simulink model "Proj4_simulink"  (R2023b)
settings: Solver=FixedStepAuto  StartTime=0.0  StopTime=10  FixedStep=0.01  RelTol=1e-3
values from neighbouring files (symbols this model uses):
  test_position = [test_position, x]    [Proj4_MainScript.m]
  test_speed = [test_speed,20]    [Proj4_MainScript.m]
  x_track = [x_straight1, x_curve1, x_straight2, x_curve2]    [Proj4_MainScript.m]
  y_track = [y_straight1, y_curve1, y_straight2, y_curve2]    [Proj4_MainScript.m]
undefined symbols (not defined in the file or in its folder): batData, carData, motorData, mph2mps
libraries: slpidlib x2
settings Model: Creator=nakro  LastModifiedBy=nakro

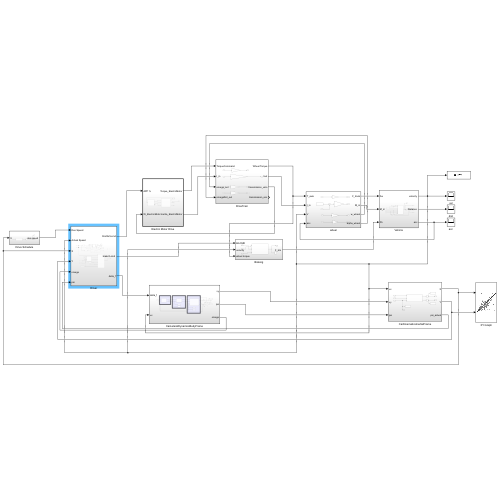
[thumbnail: Simulink's stored preview of the top-level diagram]
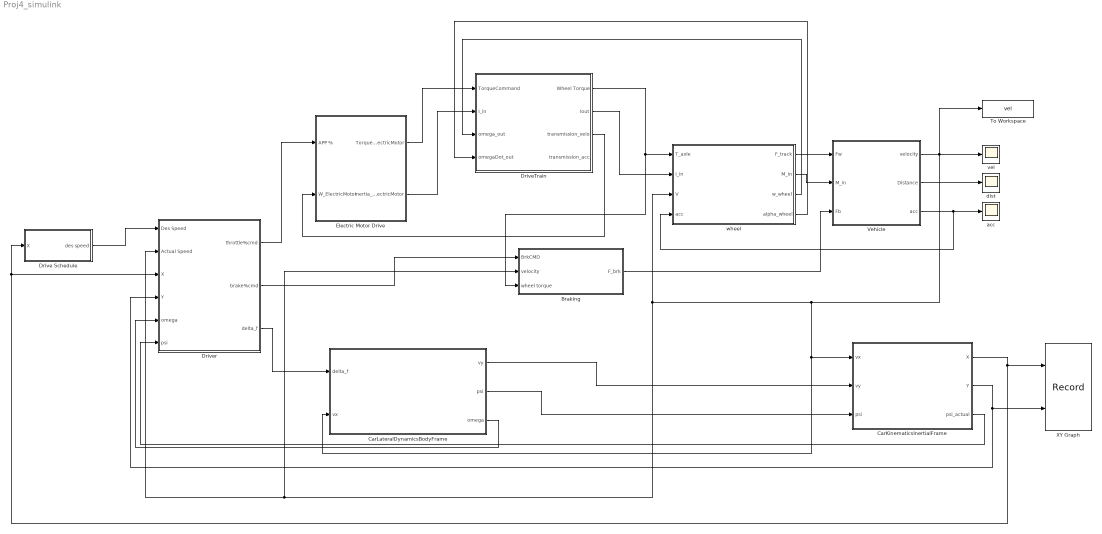
== system Proj4_simulink ==
  Braking : Subsystem
  CarKinematicsInertialFrame : Subsystem
  CarLateralDynamicsBodyFrame : Subsystem
  Drive Schedule : Subsystem
  DriveTrain : Subsystem
  "Driver " : Subsystem
  Electric Motor Drive : Subsystem  TreatAsAtomicUnit=on
  To Workspace : ToWorkspace  VariableName=vel  SaveFormat=Timeseries  SampleTime=0.01
  Vehicle : Subsystem
  XY Graph : Record  FileSettingsInternal="{\"entries\":[{\"content\":{\"excelSettings\":{\"content\":{},\"type\":\"Streamout.ExcelSettings\"}},\"type\":\"Streamout.FileSettingStorage\",\"uuid\":\"\"}],\"packageUris\":[\"http:\\/\\/schema.mathworks.com\\/mf0\\/streamout_blocks\\/R2020a\"],\"version\":\"1.0\"}"  Layout=[1 1]  SignalsInternal="{\"entries\":[{\"content\":{\"signals\":[{\"content\":{\"blockPath\":[],\"dimensions\":[1],\"domain\":\"\",\"lineColor\":\"#a2142f\",\"plots\":[1],\"port\":1,\"sid\":[\"\"],\"signalID\":43985,\"signalName\":\"CarKinematicsInertialFrame:1\"},\"type\":\"RecordBlkView.Signal\",\"uuid\":\"\"},{\"content\":{\"blockPath\":[],\"dimensions\":[1],\"domain\":\"\",\"lineColor\":\"#139fff\",\"plots\":[1],\"port\":2,\"sid\":[\"\"],\"signalID\":43989,\"signalName\":\"CarKinematicsInertialFrame:2\"},\"type\":\"RecordBlkView.Signal\",\"uuid\":\"\"}]},\"type\":\"RecordBlkView.InputSignals\",\"uuid\":\"\"}],\"packageUris\":[\"http:\\/\\/schema.mathworks.com\\/mf0\\/streamout_blocks\\/R2020a\"],\"version\":\"1.0\"}"  VisualizationBindings="{\"xyplotplugin\":{\"info\":[{\"series\":[{\"bindingParametersList\":[{\"parameter\":\"X-Axis\",\"signalID\":43985,\"signalName\":\"CarKinematicsInertialFrame:1\"},{\"parameter\":\"Y-Axis\",\"signalID\":43989,\"signalName\":\"CarKinematicsInertialFrame:2\"}],\"seriesID\":61081}],\"subplotID\":1}]}}"  CompatibilityTag=XY  st=-1
  acc : Scope
  dist : Scope
  vel : Scope
  "wheel " : Subsystem
  wires:
  CarLateralDynamicsBodyFrame/2(psi) -> CarKinematicsInertialFrame/3(psi)
  CarKinematicsInertialFrame/1(X) -> "Driver "/3(X), Drive Schedule/1(X), XY Graph/1
  CarLateralDynamicsBodyFrame/1(vy) -> CarKinematicsInertialFrame/2(vy)
  CarKinematicsInertialFrame/2(Y) -> XY Graph/2, "Driver "/4(Y)
  Electric Motor Drive/1(Torque_ElectricMotor) -> DriveTrain/1(TorqueCommand)
  Vehicle/1("velocity ") -> Braking/2("velocity "), "Driver "/2(Actual Speed), "wheel "/3(V), CarKinematicsInertialFrame/1(vx), CarLateralDynamicsBodyFrame/2(vx), To Workspace/1, vel/1
  Electric Motor Drive/2(Inertia_ElectricMotor) -> DriveTrain/2(I_in)
  "wheel "/3(w_wheel) -> DriveTrain/3(omega_out)
  "Driver "/1(throttle%cmd) -> Electric Motor Drive/1(APP %)
  "wheel "/4(alpha_wheel) -> DriveTrain/4(omegaDot_out)
  "wheel "/1(F_track) -> Vehicle/1("Fw ")
  Vehicle/2("Distance ") -> dist/1
  DriveTrain/1(Wheel Torque) -> Braking/3(wheel torque), "wheel "/1(T_axle)
  Vehicle/3(acc) -> acc/1, "wheel "/4(acc)
  DriveTrain/3(transmission_velo) -> Electric Motor Drive/2(W_ElectricMotor)
  "wheel "/2(M_in) -> Vehicle/2("M_in ")
  Braking/1("F_brk ") -> Vehicle/3("Fb ")
  Drive Schedule/1("des speed ") -> "Driver "/1("Des Speed ")
  DriveTrain/2(Iout) -> "wheel "/2(I_in)
  "Driver "/2("brake%cmd ") -> Braking/1("BrkCMD ")
  "Driver "/3(delta_f) -> CarLateralDynamicsBodyFrame/1(delta_f)
  CarKinematicsInertialFrame/3(psi_actual) -> "Driver "/6(psi)
  CarLateralDynamicsBodyFrame/3(omega) -> "Driver "/5(omega)

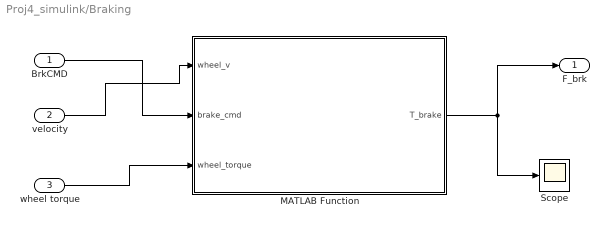
== system Proj4_simulink/Braking ==
  "BrkCMD " : Inport
  "velocity " : Inport  Port=2
  wheel torque : Inport  Port=3
  MATLAB Function : MATLAB Function  TreatAsAtomicUnit=on
  Scope : Scope
  "F_brk " : Outport  VectorParamsAs1DForOutWhenUnconnected=off
  wires:
  "BrkCMD "/1 -> MATLAB Function/2(brake_cmd)
  "velocity "/1 -> MATLAB Function/1(wheel_v)
  wheel torque/1 -> MATLAB Function/3(wheel_torque)
  MATLAB Function/1(T_brake) -> Scope/1, "F_brk "/1

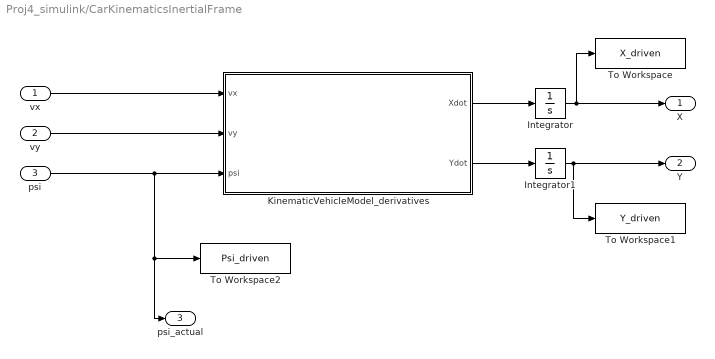
== system Proj4_simulink/CarKinematicsInertialFrame ==
  vx : Inport
  vy : Inport  Port=2
  psi : Inport  Port=3
  Integrator : Integrator  InitialCondition=carData.init.X0
  Integrator1 : Integrator  InitialCondition=carData.init.Y0
  KinematicVehicleModel_derivatives : MATLAB Function  TreatAsAtomicUnit=on  mask{obj=carData}
      mask prompts: obj "obj structure"
  To Workspace : ToWorkspace  VariableName=X_driven  SaveFormat=Timeseries  SampleTime=0.1
  To Workspace1 : ToWorkspace  VariableName=Y_driven  SaveFormat=Timeseries  SampleTime=0.1
  To Workspace2 : ToWorkspace  VariableName=Psi_driven  SaveFormat=Timeseries  SampleTime=0.1
  X : Outport
  Y : Outport  Port=2
  psi_actual : Outport  Port=3
  wires:
  KinematicVehicleModel_derivatives/1(Xdot) -> Integrator/1
  KinematicVehicleModel_derivatives/2(Ydot) -> Integrator1/1
  Integrator/1 -> To Workspace/1, X/1
  Integrator1/1 -> To Workspace1/1, Y/1
  vx/1 -> KinematicVehicleModel_derivatives/1(vx)
  vy/1 -> KinematicVehicleModel_derivatives/2(vy)
  psi/1 -> psi_actual/1, To Workspace2/1, KinematicVehicleModel_derivatives/3(psi)

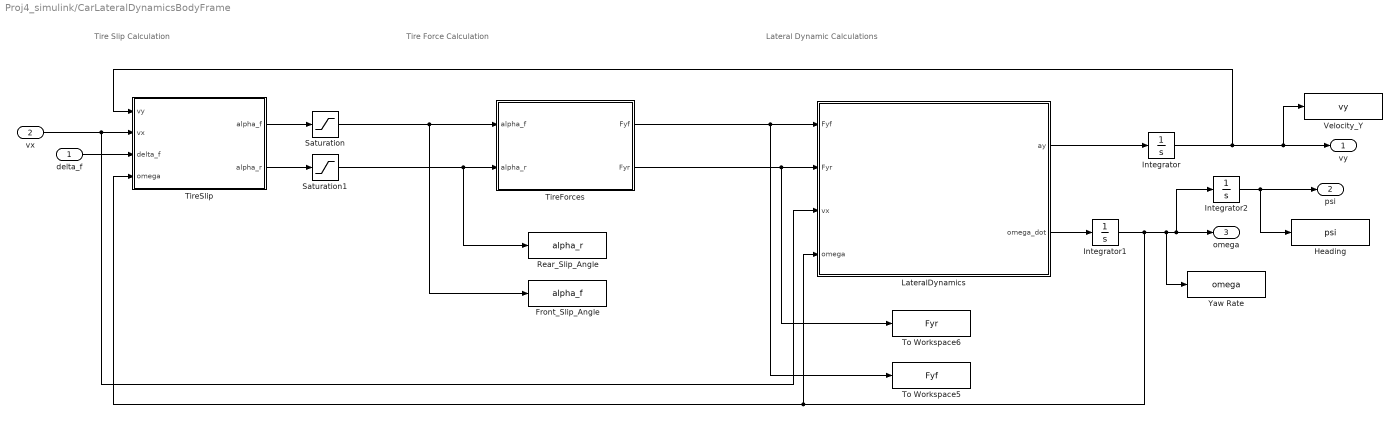
== system Proj4_simulink/CarLateralDynamicsBodyFrame ==
  note: Tire Slip Calculation
  note: Tire Force Calculation
  note: Lateral Dynamic Calculations
  delta_f : Inport
  vx : Inport  Port=2
  Front_Slip_Angle : ToWorkspace  VariableName=alpha_f  SaveFormat=Timeseries  SampleTime=0.01
  Heading : ToWorkspace  VariableName=psi  SaveFormat=Timeseries  SampleTime=0.01
  Integrator : Integrator  InitialCondition=carData.init.vy0
  Integrator1 : Integrator  InitialCondition=carData.init.omega0
  Integrator2 : Integrator  InitialCondition=carData.init.psi0
  LateralDynamics : MATLAB Function  TreatAsAtomicUnit=on  mask{obj=carData}
      mask prompts: obj "obj structure"
  Rear_Slip_Angle : ToWorkspace  VariableName=alpha_r  SaveFormat=Timeseries  SampleTime=0.01
  Saturation : Saturate  UpperLimit=carData.maxAlpha  LowerLimit=-carData.maxAlpha
  Saturation1 : Saturate  UpperLimit=carData.maxAlpha  LowerLimit=-carData.maxAlpha
  TireForces : MATLAB Function  TreatAsAtomicUnit=on  mask{obj=carData}
      mask prompts: obj "obj structure"
  TireSlip : MATLAB Function  TreatAsAtomicUnit=on  mask{obj=carData}
      mask prompts: obj "obj structure"
  To Workspace5 : ToWorkspace  VariableName=Fyf  SaveFormat=Timeseries  SampleTime=0.01
  To Workspace6 : ToWorkspace  VariableName=Fyr  SaveFormat=Timeseries  SampleTime=0.01
  Velocity_Y : ToWorkspace  VariableName=vy  SaveFormat=Timeseries  SampleTime=0.01
  Yaw Rate : ToWorkspace  VariableName=omega  SaveFormat=Timeseries  SampleTime=0.01
  vy : Outport
  psi : Outport  Port=2
  omega : Outport  Port=3
  wires:
  LateralDynamics/1(ay) -> Integrator/1
  Integrator/1 -> vy/1, Velocity_Y/1, TireSlip/1(vy)
  LateralDynamics/2(omega_dot) -> Integrator1/1
  Integrator1/1 -> Integrator2/1, omega/1, Yaw Rate/1, LateralDynamics/4(omega), TireSlip/4(omega)
  TireSlip/1(alpha_f) -> Saturation/1
  TireSlip/2(alpha_r) -> Saturation1/1
  TireForces/1(Fyf) -> LateralDynamics/1(Fyf), To Workspace5/1
  TireForces/2(Fyr) -> LateralDynamics/2(Fyr), To Workspace6/1
  Saturation/1 -> TireForces/1(alpha_f), Front_Slip_Angle/1
  Saturation1/1 -> TireForces/2(alpha_r), Rear_Slip_Angle/1
  vx/1 -> TireSlip/2(vx), LateralDynamics/3(vx)
  delta_f/1 -> TireSlip/3(delta_f)
  Integrator2/1 -> Heading/1, psi/1

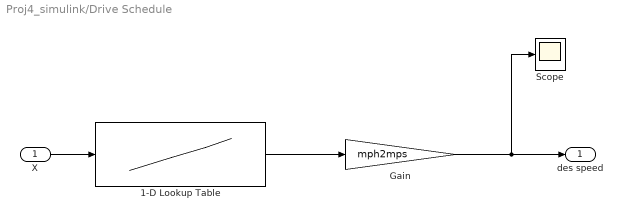
== system Proj4_simulink/Drive Schedule ==
  X : Inport
  1-D Lookup Table : Lookup_n-D  NumberOfTableDimensions=1  BreakpointsForDimension1=test_position  Table=test_speed  InternalRulePriority=Speed  RndMeth=Simplest
  Gain : Gain  Gain=mph2mps
  Scope : Scope
  "des speed " : Outport  VectorParamsAs1DForOutWhenUnconnected=off
  wires:
  1-D Lookup Table/1 -> Gain/1
  Gain/1 -> "des speed "/1, Scope/1
  X/1 -> 1-D Lookup Table/1

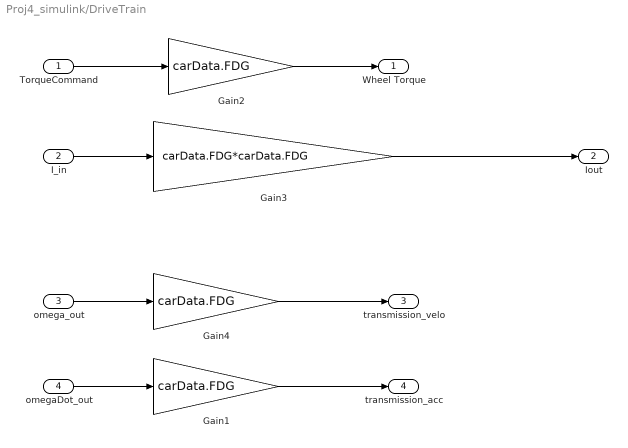
== system Proj4_simulink/DriveTrain ==
  TorqueCommand : Inport
  I_in : Inport  Port=2
  omega_out : Inport  Port=3
  omegaDot_out : Inport  Port=4
  Gain1 : Gain  Gain=carData.FDG
  Gain2 : Gain  Gain=carData.FDG
  Gain3 : Gain  Gain=carData.FDG*carData.FDG
  Gain4 : Gain  Gain=carData.FDG
  Wheel Torque : Outport
  Iout : Outport  Port=2
  transmission_velo : Outport  Port=3
  transmission_acc : Outport  Port=4
  wires:
  Gain4/1 -> transmission_velo/1
  Gain3/1 -> Iout/1
  Gain1/1 -> transmission_acc/1
  Gain2/1 -> Wheel Torque/1
  TorqueCommand/1 -> Gain2/1
  omega_out/1 -> Gain4/1
  omegaDot_out/1 -> Gain1/1
  I_in/1 -> Gain3/1

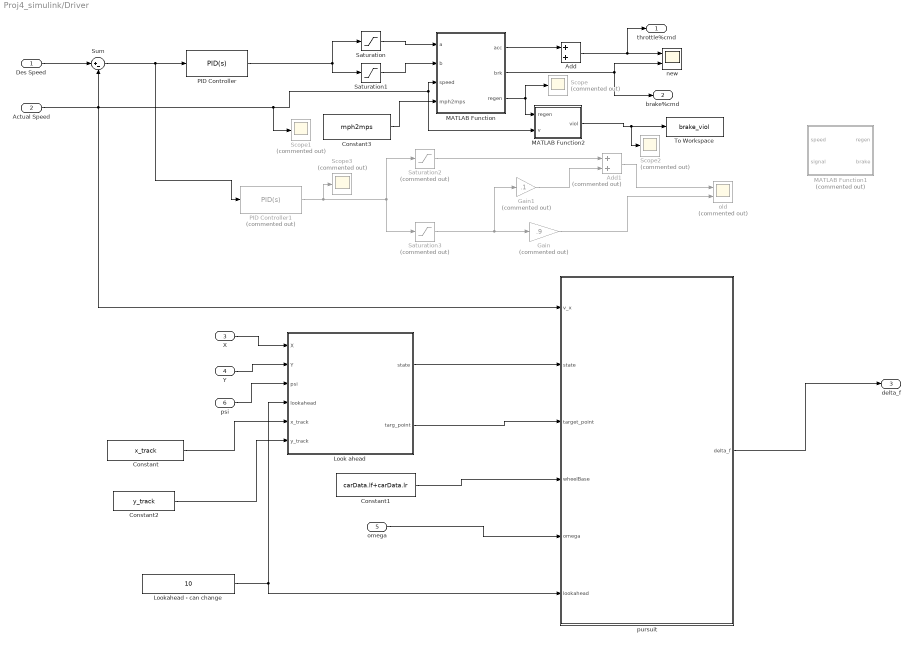
== system Proj4_simulink/Driver  ==
  "Des Speed " : Inport
  Actual Speed : Inport  Port=2
  X : Inport  Port=3
  Y : Inport  Port=4
  omega : Inport  Port=5
  psi : Inport  Port=6
  Add : Sum
  Add1 : Sum  Commented=on
  Constant : Constant  Value=x_track
  Constant1 : Constant  Value=carData.lf+carData.lr
  Constant2 : Constant  Value=y_track
  Constant3 : Constant  Value=mph2mps
  Gain : Gain  Commented=on  Gain=.9
  Gain1 : Gain  Commented=on  Gain=.1
  Look ahead : MATLAB Function  TreatAsAtomicUnit=on
  Lookahead - can change : Constant  Value=10
  MATLAB Function : MATLAB Function  TreatAsAtomicUnit=on
  MATLAB Function1 : MATLAB Function  Commented=on  TreatAsAtomicUnit=on
  MATLAB Function2 : MATLAB Function  TreatAsAtomicUnit=on
  PID Controller : slpidlib/PID Controller  Controller=PID  Form=Parallel  TimeDomain=Continuous-time  UseExternalTs=on  SampleTime=0.01  IntegratorMethod=Forward Euler  FilterMethod=Forward Euler  ControllerParametersSource=internal  P=.1  I=0  UseKiTs=off  D=0  N=100  UseFilter=on  TunerSelectOption=Transfer Function Based (PID Tuner App)  InitialConditionSource=internal  InitialConditionForIntegrator=0  InitialConditionForFilter=0  DifferentiatorICPrevScaledInput=0  ExternalReset=none  TrackingMode=off  Kt=1  LimitOutput=on  SatLimitsSource=internal  UpperSaturationLimit=1  LowerSaturationLimit=-1  LinearizeAsGain=off  AntiWindupMode=none  Kb=1  LimitIntegrator=off  UpperIntegratorSaturationLimit=inf  LowerIntegratorSaturationLimit=-inf  POutMin=[]  POutMax=[]  IOutMin=[]  IOutMax=[]  DOutMin=[]  DOutMax=[]  NOutMin=[]  NOutMax=[]  SumOutMin=[]  SumOutMax=[]  SaturationOutMin=[]  SaturationOutMax=[]  PParamMin=[]  PParamMax=[]  IParamMin=[]  IParamMax=[]  DParamMin=[]  DParamMax=[]  NParamMin=[]  NParamMax=[]  KbParamMin=[]  KbParamMax=[]  KtParamMin=[]  KtParamMax=[]  KbOutMin=[]  KbOutMax=[]  KtOutMin=[]  KtOutMax=[]  IntegratorOutMin=[]  IntegratorOutMax=[]  FilterOutMin=[]  FilterOutMax=[]  SumI1OutMin=[]  SumI1OutMax=[]  SumI2OutMin=[]  SumI2OutMax=[]  SumI3OutMin=[]  SumI3OutMax=[]  SumI4OutMin=[]  SumI4OutMax=[]  SumDOutMin=[]  SumDOutMax=[]  DifferentiatorOutMin=[]  DifferentiatorOutMax=[]  FilterDiffOutCoefMin=[]  FilterDiffOutCoefMax=[]  ReciprocalOutMin=[]  ReciprocalOutMax=[]  SumDenOutMin=[]  SumDenOutMax=[]  SumNumOutMin=[]  SumNumOutMax=[]  DivideOutMin=[]  DivideOutMax=[]  UdiffTsProdOutMin=[]  UdiffTsProdOutMax=[]  NTsProdOutMin=[]  NTsProdOutMax=[]  UintegralTsProdOutMin=[]  UintegralTsProdOutMax=[]  UngainTsProdOutMin=[]  UngainTsProdOutMax=[]  ClampingZeroOutDataTypeStr=Inherit: Inherit via back propagation  ClampingZeroOutMin=[]  ClampingZeroOutMax=[]  FilterDenConstantOutDataTypeStr=Inherit: Inherit via back propagation  FilterDenConstantOutMin=[]  FilterDenConstantOutMax=[]  PCopyOutDataTypeStr=Inherit: Inherit via back propagation  PCopyOutMin=[]  PCopyOutMax=[]  NCopyOutDataTypeStr=Inherit: Inherit via back propagation  NCopyOutMin=[]  NCopyOutMax=[]  IntegratorContinuousStateAttributes=''  IntegratorStateMustResolveToSignalObject=off  IntegratorRTWStateStorageClass=Auto  FilterContinuousStateAttributes=''  FilterStateMustResolveToSignalObject=off  FilterRTWStateStorageClass=Auto  ParallelPVariant=InternalParameters  IdealPVariant=Disabled  IVariant=InternalParameters  DVariant=InternalParameters  IntegratorVariant=Continuous  SatVariant=Enabled  AWVariant=Passthrough  PCopyVariant=Disabled  TRVariant=Disabled  FdbkBlocksVariant=Forward  IdealPFdbkVariant=Disabled  SatFdbkVariant=Disabled  DerivativeFilterVariant=ContFilter  NVariant=InternalParameters  NCopyVariant=Disabled  FilterICVariant=InternalICsFilter  IntegratorICVariant=InternalICs  ExternalResetVariant=Disabled  TRSumVariant=Passthrough  SumFdbkVariant=Disabled  SumVariant=Sum_PID  TsampFilterVariant=InternalTs  TsampNgainVariant=Passthrough  TsampIntegralVariant=Disabled_SignalSpec  ExternalSaturationOutDataTypeStr=Inherit: Same as second input
  PID Controller1 : slpidlib/PID Controller  Commented=on  Controller=PID  Form=Parallel  TimeDomain=Continuous-time  UseExternalTs=off  SampleTime=-1  IntegratorMethod=Forward Euler  FilterMethod=Forward Euler  ControllerParametersSource=internal  P=.1  I=0  UseKiTs=off  D=0  N=100  UseFilter=on  TunerSelectOption=Transfer Function Based (PID Tuner App)  InitialConditionSource=internal  InitialConditionForIntegrator=0  InitialConditionForFilter=0  DifferentiatorICPrevScaledInput=0  ExternalReset=none  TrackingMode=off  Kt=1  LimitOutput=on  SatLimitsSource=internal  UpperSaturationLimit=1  LowerSaturationLimit=-1  LinearizeAsGain=off  AntiWindupMode=none  Kb=1  LimitIntegrator=off  UpperIntegratorSaturationLimit=inf  LowerIntegratorSaturationLimit=-inf  POutMin=[]  POutMax=[]  IOutMin=[]  IOutMax=[]  DOutMin=[]  DOutMax=[]  NOutMin=[]  NOutMax=[]  SumOutMin=[]  SumOutMax=[]  SaturationOutMin=[]  SaturationOutMax=[]  PParamMin=[]  PParamMax=[]  IParamMin=[]  IParamMax=[]  DParamMin=[]  DParamMax=[]  NParamMin=[]  NParamMax=[]  KbParamMin=[]  KbParamMax=[]  KtParamMin=[]  KtParamMax=[]  KbOutMin=[]  KbOutMax=[]  KtOutMin=[]  KtOutMax=[]  IntegratorOutMin=[]  IntegratorOutMax=[]  FilterOutMin=[]  FilterOutMax=[]  SumI1OutMin=[]  SumI1OutMax=[]  SumI2OutMin=[]  SumI2OutMax=[]  SumI3OutMin=[]  SumI3OutMax=[]  SumI4OutMin=[]  SumI4OutMax=[]  SumDOutMin=[]  SumDOutMax=[]  DifferentiatorOutMin=[]  DifferentiatorOutMax=[]  FilterDiffOutCoefMin=[]  FilterDiffOutCoefMax=[]  ReciprocalOutMin=[]  ReciprocalOutMax=[]  SumDenOutMin=[]  SumDenOutMax=[]  SumNumOutMin=[]  SumNumOutMax=[]  DivideOutMin=[]  DivideOutMax=[]  UdiffTsProdOutMin=[]  UdiffTsProdOutMax=[]  NTsProdOutMin=[]  NTsProdOutMax=[]  UintegralTsProdOutMin=[]  UintegralTsProdOutMax=[]  UngainTsProdOutMin=[]  UngainTsProdOutMax=[]  ClampingZeroOutDataTypeStr=Inherit: Inherit via back propagation  ClampingZeroOutMin=[]  ClampingZeroOutMax=[]  FilterDenConstantOutDataTypeStr=Inherit: Inherit via back propagation  FilterDenConstantOutMin=[]  FilterDenConstantOutMax=[]  PCopyOutDataTypeStr=Inherit: Inherit via back propagation  PCopyOutMin=[]  PCopyOutMax=[]  NCopyOutDataTypeStr=Inherit: Inherit via back propagation  NCopyOutMin=[]  NCopyOutMax=[]  IntegratorContinuousStateAttributes=''  IntegratorStateMustResolveToSignalObject=off  IntegratorRTWStateStorageClass=Auto  FilterContinuousStateAttributes=''  FilterStateMustResolveToSignalObject=off  FilterRTWStateStorageClass=Auto  ParallelPVariant=InternalParameters  IdealPVariant=Disabled  IVariant=InternalParameters  DVariant=InternalParameters  IntegratorVariant=Continuous  SatVariant=Enabled  AWVariant=Passthrough  PCopyVariant=Disabled  TRVariant=Disabled  FdbkBlocksVariant=Forward  IdealPFdbkVariant=Disabled  SatFdbkVariant=Disabled  DerivativeFilterVariant=ContFilter  NVariant=InternalParameters  NCopyVariant=Disabled  FilterICVariant=InternalICsFilter  IntegratorICVariant=InternalICs  ExternalResetVariant=Disabled  TRSumVariant=Passthrough  SumFdbkVariant=Disabled  SumVariant=Sum_PID  TsampFilterVariant=InternalTs  TsampNgainVariant=Passthrough  TsampIntegralVariant=Disabled_SignalSpec  ExternalSaturationOutDataTypeStr=Inherit: Same as second input
  Saturation : Saturate  UpperLimit=1  LowerLimit=0
  Saturation1 : Saturate  UpperLimit=0  LowerLimit=-1
  Saturation2 : Saturate  Commented=on  UpperLimit=1  LowerLimit=0
  Saturation3 : Saturate  Commented=on  UpperLimit=0  LowerLimit=-1
  Scope{,1..3} (4 alike) : Scope  Commented=on
  Sum : Sum  Inputs=|+-
  To Workspace : ToWorkspace  VariableName=brake_viol  SaveFormat=Timeseries  SampleTime=0.01
  new : Scope  NumInputPorts=2
  old : Scope  Commented=on  NumInputPorts=2
  pursuit : MATLAB Function  TreatAsAtomicUnit=on
  throttle%cmd : Outport
  "brake%cmd " : Outport  Port=2
  delta_f : Outport  Port=3
  wires:
  Sum/1 -> PID Controller/1, PID Controller1/1
  PID Controller/1 -> Saturation1/1, Saturation/1
  Saturation1/1 -> MATLAB Function/2(b)
  Saturation/1 -> MATLAB Function/1(a)
  MATLAB Function/2(brk) -> "brake%cmd "/1, new/2
  Look ahead/1(state) -> pursuit/2(state)
  Look ahead/2(targ_point) -> pursuit/3(target_point)
  Constant1/1 -> pursuit/4(wheelBase)
  omega/1 -> pursuit/5(omega)
  Lookahead - can change/1 -> Look ahead/4(lookahead), pursuit/6(lookahead)
  Y/1 -> Look ahead/2(Y)
  X/1 -> Look ahead/1(X)
  psi/1 -> Look ahead/3(psi)
  Constant/1 -> Look ahead/5(x_track)
  Constant2/1 -> Look ahead/6(y_track)
  pursuit/1(delta_f) -> delta_f/1
  MATLAB Function/1(acc) -> Add/1
  Add/1 -> throttle%cmd/1, new/1
  "Des Speed "/1 -> Sum/1
  Add1/1 -> old/1
  Gain/1 -> old/2
  Saturation3/1 -> Gain1/1, Gain/1
  Gain1/1 -> Add1/2
  PID Controller1/1 -> Scope3/1, Saturation3/1, Saturation2/1
  Saturation2/1 -> Add1/1
  Constant3/1 -> MATLAB Function/4(mph2mps)
  MATLAB Function2/1(viol) -> Scope2/1, To Workspace/1
  MATLAB Function/3(regen) -> Scope/1, MATLAB Function2/1(regen)
  Actual Speed/1 -> Sum/2, Scope1/1, MATLAB Function2/2(v), MATLAB Function/3(speed), pursuit/1(v_x)

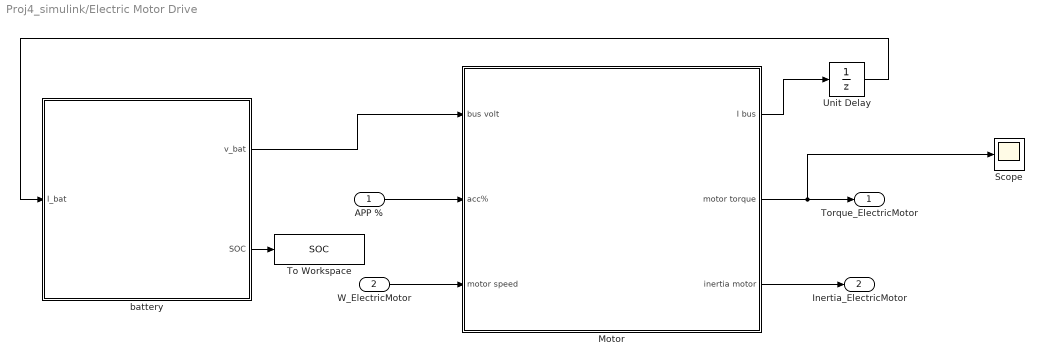
== system Proj4_simulink/Electric Motor Drive ==
  APP % : Inport
  W_ElectricMotor : Inport  Port=2
  Motor : Subsystem  TreatAsAtomicUnit=on
  Scope : Scope
  To Workspace : ToWorkspace  VariableName=SOC  SaveFormat=Timeseries  SampleTime=0.01
  Unit Delay : UnitDelay  SampleTime=-1  HasFrameUpgradeWarning=on
  battery : Subsystem  TreatAsAtomicUnit=on
  Torque_ElectricMotor : Outport
  Inertia_ElectricMotor : Outport  Port=2
  wires:
  Motor/3(inertia motor) -> Inertia_ElectricMotor/1
  APP %/1 -> Motor/2(acc%)
  W_ElectricMotor/1 -> Motor/3(motor speed)
  battery/1(v_bat) -> Motor/1(bus volt)
  Motor/1(I bus) -> Unit Delay/1
  Unit Delay/1 -> battery/1(I_bat)
  Motor/2(motor torque) -> Scope/1, Torque_ElectricMotor/1
  battery/2(SOC) -> To Workspace/1

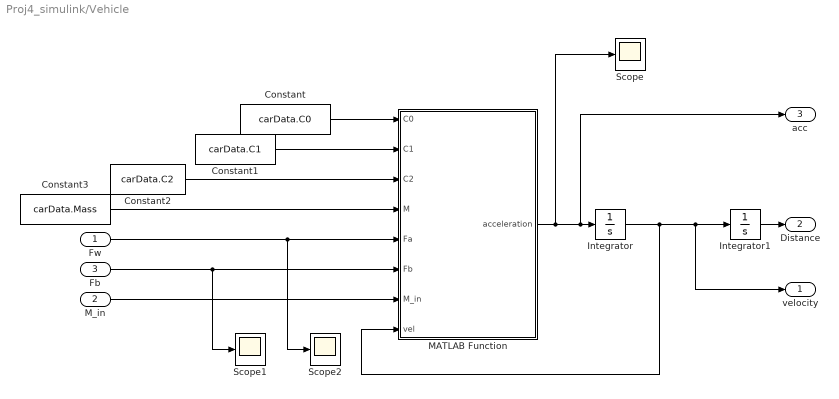
== system Proj4_simulink/Vehicle ==
  "Fw " : Inport
  "M_in " : Inport  Port=2
  "Fb " : Inport  Port=3
  Constant : Constant  Value=carData.C0
  Constant1 : Constant  Value=carData.C1
  Constant2 : Constant  Value=carData.C2
  Constant3 : Constant  Value=carData.Mass
  Integrator : Integrator  LimitOutput=on  LowerSaturationLimit=0
  Integrator1 : Integrator
  MATLAB Function : MATLAB Function  TreatAsAtomicUnit=on
  Scope : Scope
  Scope1 : Scope
  Scope2 : Scope
  "velocity " : Outport  VectorParamsAs1DForOutWhenUnconnected=off
  "Distance " : Outport  Port=2  VectorParamsAs1DForOutWhenUnconnected=off
  acc : Outport  Port=3
  wires:
  Constant1/1 -> MATLAB Function/2(C1)
  Constant/1 -> MATLAB Function/1(C0)
  MATLAB Function/1(acceleration) -> Scope/1, acc/1, Integrator/1
  Constant2/1 -> MATLAB Function/3(C2)
  Constant3/1 -> MATLAB Function/4(M)
  Integrator/1 -> MATLAB Function/8(vel), "velocity "/1, Integrator1/1
  Integrator1/1 -> "Distance "/1
  "M_in "/1 -> MATLAB Function/7(M_in)
  "Fw "/1 -> MATLAB Function/5(Fa), Scope2/1
  "Fb "/1 -> Scope1/1, MATLAB Function/6(Fb)

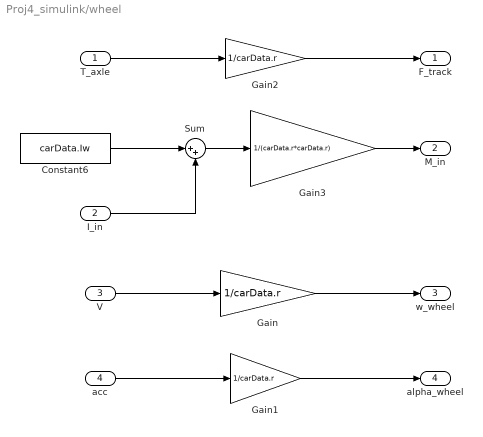
== system Proj4_simulink/wheel  ==
  T_axle : Inport
  I_in : Inport  Port=2
  V : Inport  Port=3
  acc : Inport  Port=4
  Constant6 : Constant  Value=carData.Iw
  Gain : Gain  Gain=1/carData.r
  Gain1 : Gain  Gain=1/carData.r
  Gain2 : Gain  Gain=1/carData.r
  Gain3 : Gain  Gain=1/(carData.r*carData.r)
  Sum : Sum  Inputs=|++
  F_track : Outport
  M_in : Outport  Port=2
  w_wheel : Outport  Port=3
  alpha_wheel : Outport  Port=4
  wires:
  Gain/1 -> w_wheel/1
  V/1 -> Gain/1
  acc/1 -> Gain1/1
  Gain1/1 -> alpha_wheel/1
  T_axle/1 -> Gain2/1
  Gain2/1 -> F_track/1
  Gain3/1 -> M_in/1
  Constant6/1 -> Sum/1
  I_in/1 -> Sum/2
  Sum/1 -> Gain3/1

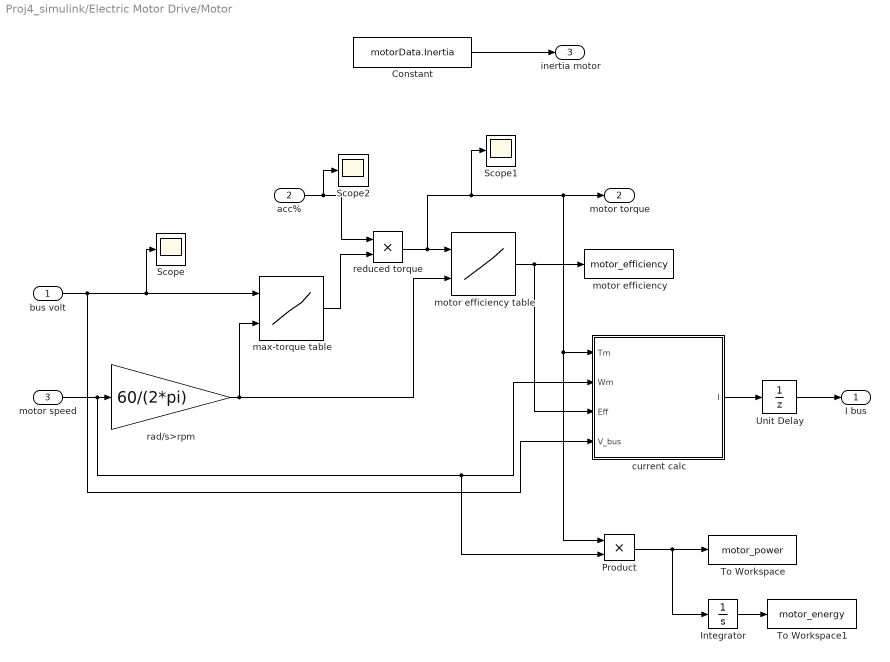
== system Proj4_simulink/Electric Motor Drive/Motor ==
  bus volt : Inport
  acc% : Inport  Port=2
  motor speed : Inport  Port=3
  Constant : Constant  Value=motorData.Inertia
  Integrator : Integrator
  Product : Product
  Scope : Scope
  Scope1 : Scope
  Scope2 : Scope
  To Workspace : ToWorkspace  VariableName=motor_power  SaveFormat=Timeseries  SampleTime=0.01
  To Workspace1 : ToWorkspace  VariableName=motor_energy  SaveFormat=Timeseries  SampleTime=0.01
  Unit Delay : UnitDelay  SampleTime=-1  HasFrameUpgradeWarning=on
  current calc : MATLAB Function  TreatAsAtomicUnit=on
  max-torque table : Lookup_n-D  BreakpointsForDimension1=motorData.vbus  BreakpointsForDimension2=motorData.rpm  BreakpointsForDimension3=[5, 7]  Table=motorData.maxtorque  InternalRulePriority=Speed  RndMeth=Simplest
      settings: InputPortMap=u0,u1
  motor efficiency : ToWorkspace  VariableName=motor_efficiency  SaveFormat=Timeseries  SampleTime=0.01
  motor efficiency table : Lookup_n-D  BreakpointsForDimension1=motorData.eta_torque  BreakpointsForDimension2=motorData.eta_speed  BreakpointsForDimension3=[5, 7]  Table=motorData.eta_val  InternalRulePriority=Speed  RndMeth=Simplest
      settings: InputPortMap=u0,u1
  rad/s>rpm : Gain  Gain=60/(2*pi)
  reduced torque : Product
  I bus : Outport
  motor torque : Outport  Port=2
  inertia motor : Outport  Port=3
  wires:
  motor speed/1 -> rad/s>rpm/1, current calc/2(Wm), Product/2
  rad/s>rpm/1 -> max-torque table/2, motor efficiency table/2
  bus volt/1 -> Scope/1, max-torque table/1, current calc/4(V_bus)
  acc%/1 -> Scope2/1, reduced torque/1
  max-torque table/1 -> reduced torque/2
  reduced torque/1 -> Scope1/1, motor torque/1, current calc/1(Tm), Product/1, motor efficiency table/1
  motor efficiency table/1 -> motor efficiency/1, current calc/3(Eff)
  Constant/1 -> inertia motor/1
  current calc/1(I) -> Unit Delay/1
  Unit Delay/1 -> I bus/1
  Product/1 -> To Workspace/1, Integrator/1
  Integrator/1 -> To Workspace1/1

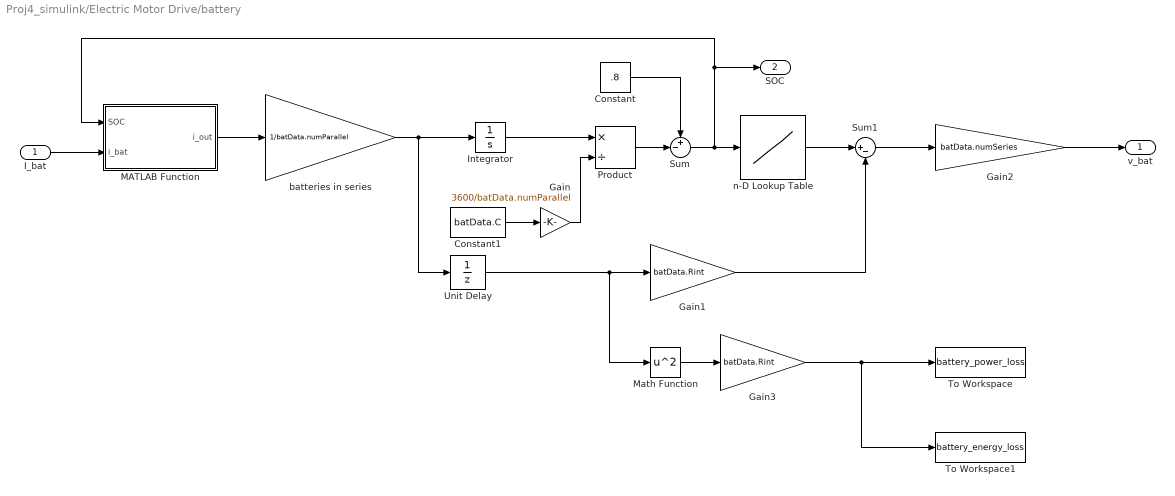
== system Proj4_simulink/Electric Motor Drive/battery ==
  I_bat : Inport
  Constant : Constant  Value=.8
  Constant1 : Constant  Value=batData.C
  Gain : Gain  Gain=3600/batData.numParallel
  Gain1 : Gain  Gain=batData.Rint
  Gain2 : Gain  Gain=batData.numSeries
  Gain3 : Gain  Gain=batData.Rint
  Integrator : Integrator
  MATLAB Function : MATLAB Function  TreatAsAtomicUnit=on
  Math Function : Math  Operator=square
  Product : Product  Inputs=*/
  Sum : Sum  Inputs=+-|
  Sum1 : Sum  Inputs=|+-
  To Workspace : ToWorkspace  VariableName=battery_power_loss  SaveFormat=Timeseries  SampleTime=0.01
  To Workspace1 : ToWorkspace  VariableName=battery_energy_loss  SaveFormat=Timeseries  SampleTime=0.01
  Unit Delay : UnitDelay  SampleTime=-1  HasFrameUpgradeWarning=on
  batteries in series : Gain  Gain=1/batData.numParallel
  n-D Lookup Table : Lookup_n-D  NumberOfTableDimensions=1  BreakpointsForDimension1=batData.SOC  BreakpointsForDimension3=[5, 7]  Table=batData.OCV  InternalRulePriority=Speed  RndMeth=Simplest
  v_bat : Outport
  SOC : Outport  Port=2
  wires:
  batteries in series/1 -> Integrator/1, Unit Delay/1
  Integrator/1 -> Product/1
  Gain/1 -> Product/2
  Product/1 -> Sum/2
  Constant/1 -> Sum/1
  Sum/1 -> n-D Lookup Table/1, MATLAB Function/1(SOC), SOC/1
  n-D Lookup Table/1 -> Sum1/1
  Unit Delay/1 -> Gain1/1, Math Function/1
  Gain1/1 -> Sum1/2
  Sum1/1 -> Gain2/1
  Gain2/1 -> v_bat/1
  Constant1/1 -> Gain/1
  Math Function/1 -> Gain3/1
  Gain3/1 -> To Workspace1/1, To Workspace/1
  I_bat/1 -> MATLAB Function/2(i_bat)
  MATLAB Function/1(i_out) -> batteries in series/1

== matlab function Proj4_simulink/Driver /MATLAB Function ==
  data: a input; acc output; b input; speed input; brk output; regen output; mph2mps input
function [acc, brk, regen]= fcn(a,b,speed,mph2mps)
mph2mps = 1;
if speed < 5/mph2mps
    regen = 0;
    acc = a;
    brk = b;
elseif speed == 25/mph2mps
    regen = 0.95;
    friction = 0.05;
    acc = a + b*regen;
    brk = b*friction;
elseif speed > 25/mph2mps
     regen = 0.95;
    friction = 0.05;
    acc = a + b*regen;
    brk = b*friction;
else
    regen = ((0.95/20)*speed) - 0.2375;
    friction = 1-regen;
    acc = a * b*regen;
    brk = b*friction;
end

== matlab function Proj4_simulink/Driver /Look ahead ==
  data: X input; state output; Y input; psi input; lookahead input; targ_point output; x_track input; y_track input
function [state, targ_point] = fcn(X, Y, psi, lookahead, x_track, y_track)

    ref = [x_track, y_track];

    state = [X, Y, psi];

    id_xy = 1:2;

    id = lookahead;

    distance = vecnorm(ref(:, id_xy)' - state(id_xy)');
    [~, min_index] = min(distance);

    for i = min_index:length(ref)
        dist = norm(ref(i, id_xy) - state(:, id_xy));
        if dist > id 
            break;
        end
    end

    targ_point = ref(i, :);

end

== matlab function Proj4_simulink/Electric Motor Drive/battery/MATLAB Function ==
  data: SOC input; i_out output; i_bat input
function i_out = fcn(SOC, i_bat)

if SOC >= .95
    i_out = 0;
elseif SOC <= .1
    i_out = 0;
else
    i_out = i_bat;

end

== matlab function Proj4_simulink/Driver /MATLAB Function1 ==
  data: regen output; speed input; signal input; brake output
function [regen, brake] = fnc(speed, signal) 

mph2mps = 0.444444;


if speed < 5/mph2mps
    mult = 0;
   
elseif speed == 25/mph2mps
    mult = 0.95;
    
elseif speed > 25/mph2mps
     mult = 0.95;
    
else
    mult = ((0.95/20)*speed) - 0.2375;
    
end

regen = mult*signal;
brake = signal - regen;

== matlab function Proj4_simulink/Driver /MATLAB Function2 ==
  data: regen input; viol output; v input
function viol = violfcn(regen, v)
    %speed = (3600/1600)*v;
    speed = v;        
    if speed < 5
        regen_vio = 0;
        if regen == regen_vio
            viol = 0;
        else
            viol = 1;
        end

    elseif speed == 25
        regen_vio = 0.95;
        if regen == regen_vio
            viol = 0;
        else
            viol = 1;
        end

    elseif v > 25
        regen_vio = 0.95;
        if regen == regen_vio
            viol = 0;
        else
            viol = 1;
        end
    else
        regen_vio = ((0.95/20)*speed) - 0.2375;
        if regen == regen_vio
            viol = 0;
        else
            viol = 1;
        end
    end

== matlab function Proj4_simulink/CarLateralDynamicsBodyFrame/LateralDynamics ==
  data: Fyf input; Fyr input size=1; vx input; omega input; ay output; obj parameter; omega_dot output
function [ay, omega_dot] = fcn(Fyf, Fyr, vx, omega, obj)

Fy = Fyf + Fyr;
ay = Fy / obj.Mass - omega * vx;
        
M = Fyf * obj.lf - Fyr * obj.lr;        
omega_dot = M / obj.Inertia;        

end

== matlab function Proj4_simulink/Driver /pursuit ==
  data: v_x input; state input; delta_f output; target_point input; wheelBase input; omega input; lookahead input
% function delta_f   = latControl(vx,X,Y,wheelBase, underSteerCoefficient)
% 
% track_radius = 200;
% track_length = 900;
% 
% track_seg1_x0 = 0;
% track_seg1_y0 = 0;
% track_seg1_x1 = track_length;
% track_seg1_y1 = 0;
% track_seg2_x0 = track_seg1_x1;
% track_seg2_y0 = track_seg1_y1;
% track_seg2_x1 = track_seg2_x0;
% track_seg2_y1 = track_seg2_y0 + 2 * track_radius;
% track_seg3_x0 = track_seg2_x1;
% track_seg3_y0 = track_seg2_y1;
% track_seg3_x1 = track_seg3_x0 - track_length;
% track_seg3_y1 = track_seg3_y0;
% track_seg4_x0 = track_seg3_x1;
% track_seg4_y0 = track_seg3_y1;
% track_seg4_x1 = track_seg1_x0;
% track_seg4_y1 = track_seg1_y0;
% 
% 
% if X > track_seg1_x0
%     if X > track_seg1_x1
%         segment = 2;
%     else
%         if Y > (track_seg2_y0 + track_seg2_y1)/2
%             segment = 3;
%         else
%             segment = 1;
%         end
%     end
% else
%     segment = 4;
% end
% 
% 
% 
% switch(segment)
%     case 1
%         delta_f = 0;
%     case 2
%         delta_f = (wheelBase / track_radius + 1 * underSteerCoefficient * vx^2);
%     case 3
%         delta_f = 0;
%     case 4
%         delta_f = (wheelBase / track_radius + 1 * underSteerCoefficient * vx^2);
%     otherwise
%         delta_f = 0;
% end
% 

function delta_f = latControl(v_x, state, target_point, wheelBase, omega, lookahead)

    current_X = state(1);
    current_Y = state(2);
    current_psi = state(3);

    targ_X = target_point(1);
    targ_Y = target_point(2);


    alpha = atan2(targ_Y - current_Y, targ_X - current_X) - current_psi;
    psi_dot_d = (2 * wheelBase * sin(alpha)) / lookahead;
    delta_f = atan(psi_dot_d);
    
end

== matlab function Proj4_simulink/CarKinematicsInertialFrame/KinematicVehicleModel_derivatives ==
  data: vx input; vy input; psi input size=1; Xdot output; Ydot output
function [Xdot, Ydot] = fcn(vx, vy, psi)
    temp = TF(psi) * [vx;vy]; 
    Xdot = temp(1);
    Ydot = temp(2);
  
end

function y = TF(psi)
    y = [cos(psi), -sin(psi); sin(psi), cos(psi)];
end

== matlab function Proj4_simulink/Braking/MATLAB Function ==
  data: wheel_v input; T_brake output; brake_cmd input; wheel_torque input
function T_brake = fcn(wheel_v, brake_cmd, wheel_torque)

if wheel_v == 0
    T_brake = -min(abs(wheel_torque), brake_cmd*10000*(wheel_torque/abs(wheel_torque) + 0.001));
else
    T_brake = -brake_cmd*10000*(wheel_v/abs(wheel_v) + 0.001);
end

== matlab function Proj4_simulink/Electric Motor Drive/Motor/current calc ==
  data: Tm input; I output; Wm input; Eff input; V_bus input
function I = fcn(Tm, Wm, Eff, V_bus)
    Pm = Tm * Wm;
    sgn_m = sign(Pm);
    Pe = Pm * (Eff^sgn_m);
    I = Pe / V_bus;
end

== matlab function Proj4_simulink/CarLateralDynamicsBodyFrame/TireSlip ==
  data: vy input size=1; vx input; delta_f input size=1; omega input; alpha_f output; obj parameter; alpha_r output
function [alpha_f, alpha_r] = fcn(vy,  vx, delta_f, omega, obj)


if abs(vx)> obj.vx_threshold1
      alpha_f = delta_f - (vy + omega * obj.lf) / vx;
      alpha_r = - (vy - omega * obj.lr) / vx;
else
      alpha_f = 0;
      alpha_r = 0;
end



end

== matlab function Proj4_simulink/CarLateralDynamicsBodyFrame/TireForces ==
  data: alpha_f input; alpha_r input; Fyf output; obj parameter; Fyr output
function [Fyf, Fyr] = fcn(alpha_f, alpha_r, obj)

Fyf = min(obj.Fyfmax,obj.Calpha_f * alpha_f);
Fyr = min(obj.Fyrmax, obj.Calpha_r * alpha_r);
end

== matlab function Proj4_simulink/Vehicle/MATLAB Function ==
  data: C0 input; acceleration output; C1 input; C2 input; M input; Fa input; Fb input; M_in input; vel input
function acceleration   = vehicle(C0,C1,C2,M,Fa,Fb,M_in, vel)

acceleration = ((Fa-Fb)-(C0+ C1*vel + C2*(vel)^2))/(M+M_in);
%acceleration = (Fa - Fb) / (M+M_in)
